simulink model "BlokRegulatoraPIDUlamkowegoRzedu"  (R2017b)
settings: Solver=VariableStepAuto  StartTime=0.0  StopTime=400  FixedStep=0.01  RelTol=1e-3  EnableMultiTasking=on
settings Model: Creator=Kuba  LastModifiedBy=Kuba
settings SolverCC: AutoInsertRateTranBlk=on
settings ConfigComp: PLC_OutputDir=Out  PLC_TargetIDE=tiaportal  PLC_GenerateReport=off  PLC_LaunchReport=off

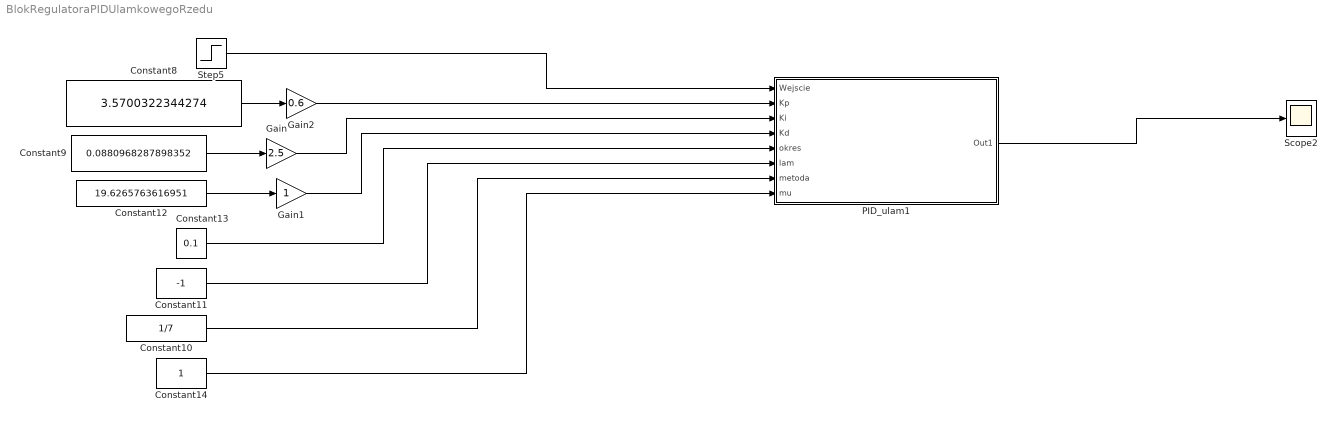
== system BlokRegulatoraPIDUlamkowegoRzedu ==
  Constant10 : Constant  Value=1/7  SampleTime=0.05
  Constant11 : Constant  Value=-1  SampleTime=0.05
  Constant12 : Constant  Value=19.6265763616951  SampleTime=0.05
  Constant13 : Constant  Value=0.1  SampleTime=0.05
  Constant14 : Constant  SampleTime=0.05
  Constant8 : Constant  Value=3.5700322344274  SampleTime=0.05
  Constant9 : Constant  Value=0.0880968287898352  SampleTime=0.05
  Gain : Gain  Gain=2.5
  Gain1 : Gain
  Gain2 : Gain  Gain=0.6
  PID_ulam1 : Subsystem  TreatAsAtomicUnit=on  SystemSampleTime=0.1
  Scope2 : Scope
  Step5 : Step  SampleTime=0.05
  wires:
  Constant10/1 -> PID_ulam1/7(metoda)
  Constant11/1 -> PID_ulam1/6(lam)
  Constant8/1 -> Gain2/1
  Constant13/1 -> PID_ulam1/5(okres)
  Constant14/1 -> PID_ulam1/8("mu ")
  Constant12/1 -> Gain1/1
  Constant9/1 -> Gain/1
  Gain/1 -> PID_ulam1/3("Ki ")
  Gain1/1 -> PID_ulam1/4("Kd ")
  Gain2/1 -> PID_ulam1/2(Kp)
  Step5/1 -> PID_ulam1/1(Wejscie)
  PID_ulam1/1(Out1) -> Scope2/1

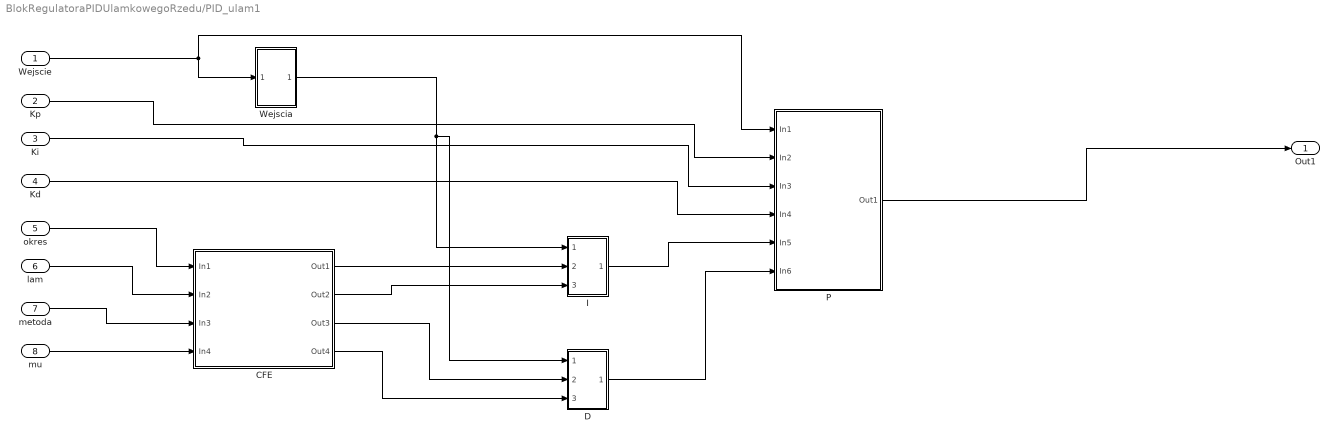
== system BlokRegulatoraPIDUlamkowegoRzedu/PID_ulam1 ==
  Wejscie : Inport
  Kp : Inport  Port=2
  "Ki " : Inport  Port=3
  "Kd " : Inport  Port=4
  okres : Inport  Port=5
  lam : Inport  Port=6
  metoda : Inport  Port=7
  "mu " : Inport  Port=8
  CFE : Subsystem  TreatAsAtomicUnit=on  SystemSampleTime=0.1
  "D " : Subsystem  TreatAsAtomicUnit=on  SystemSampleTime=0.1
  "I " : Subsystem  TreatAsAtomicUnit=on  SystemSampleTime=0.1
  "P " : Subsystem  TreatAsAtomicUnit=on  SystemSampleTime=0.1
  Wejscia : Subsystem  TreatAsAtomicUnit=on  SystemSampleTime=0.1
  Out1 : Outport
  wires:
  lam/1 -> CFE/2(In2)
  okres/1 -> CFE/1(In1)
  metoda/1 -> CFE/3(In3)
  "mu "/1 -> CFE/4(In4)
  Wejscie/1 -> "P "/1(In1), Wejscia/1(In1)
  Wejscia/1(Out1) -> "I "/1(In1), "D "/1(In1)
  CFE/3(Out3) -> "D "/2(In2)
  CFE/4(Out4) -> "D "/3(In3)
  CFE/1(Out1) -> "I "/2(In2)
  CFE/2(Out2) -> "I "/3(In3)
  Kp/1 -> "P "/2(In2)
  "Ki "/1 -> "P "/3(In3)
  "Kd "/1 -> "P "/4(In4)
  "I "/1(Out1) -> "P "/5(In5)
  "D "/1(Out1) -> "P "/6(In6)
  "P "/1(Out1) -> Out1/1

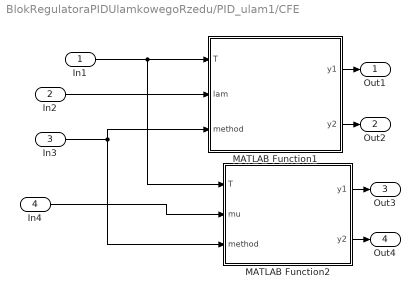
== system BlokRegulatoraPIDUlamkowegoRzedu/PID_ulam1/CFE ==
  In1 : Inport
  In2 : Inport  Port=2
  In3 : Inport  Port=3
  In4 : Inport  Port=4
  MATLAB Function1 : MATLAB Function  TreatAsAtomicUnit=on
  MATLAB Function2 : MATLAB Function  TreatAsAtomicUnit=on
  Out1 : Outport
  Out2 : Outport  Port=2
  Out3 : Outport  Port=3
  Out4 : Outport  Port=4
  wires:
  In1/1 -> MATLAB Function2/1(T), MATLAB Function1/1(T)
  In2/1 -> MATLAB Function1/2(lam)
  In3/1 -> MATLAB Function1/3(method), MATLAB Function2/3(method)
  In4/1 -> MATLAB Function2/2(mu)
  MATLAB Function1/1(y1) -> Out1/1
  MATLAB Function2/1(y1) -> Out3/1
  MATLAB Function1/2(y2) -> Out2/1
  MATLAB Function2/2(y2) -> Out4/1

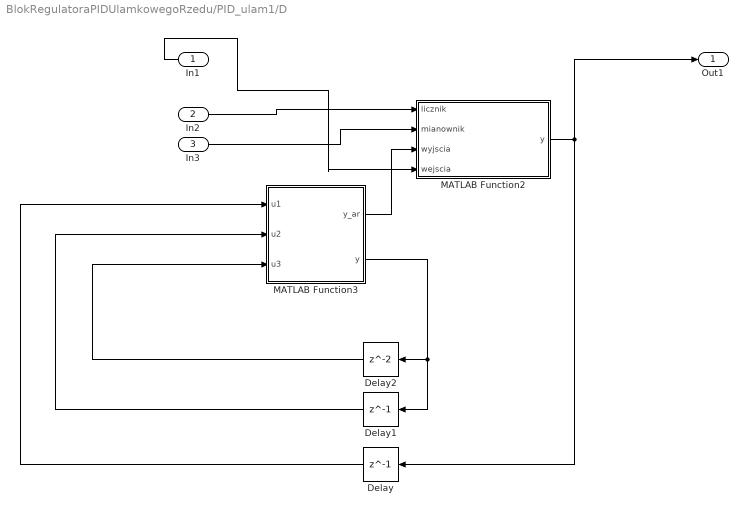
== system BlokRegulatoraPIDUlamkowegoRzedu/PID_ulam1/D  ==
  In1 : Inport
  In2 : Inport  Port=2
  In3 : Inport  Port=3
  Delay : Delay  DelayLength=1  SampleTime=0.1
  Delay1 : Delay  DelayLength=1  SampleTime=0.1
  Delay2 : Delay  SampleTime=0.1
  MATLAB Function2 : MATLAB Function  TreatAsAtomicUnit=on  SystemSampleTime=0.1
  MATLAB Function3 : MATLAB Function  TreatAsAtomicUnit=on  SystemSampleTime=0.1
  Out1 : Outport
  wires:
  In3/1 -> MATLAB Function2/2(mianownik)
  In2/1 -> MATLAB Function2/1(licznik)
  In1/1 -> MATLAB Function2/4(wejscia)
  Delay1/1 -> MATLAB Function3/2(u2)
  MATLAB Function3/2(y) -> Delay2/1, Delay1/1
  MATLAB Function3/1(y_ar) -> MATLAB Function2/3(wyjscia)
  Delay/1 -> MATLAB Function3/1(u1)
  MATLAB Function2/1(y) -> Out1/1, Delay/1
  Delay2/1 -> MATLAB Function3/3(u3)

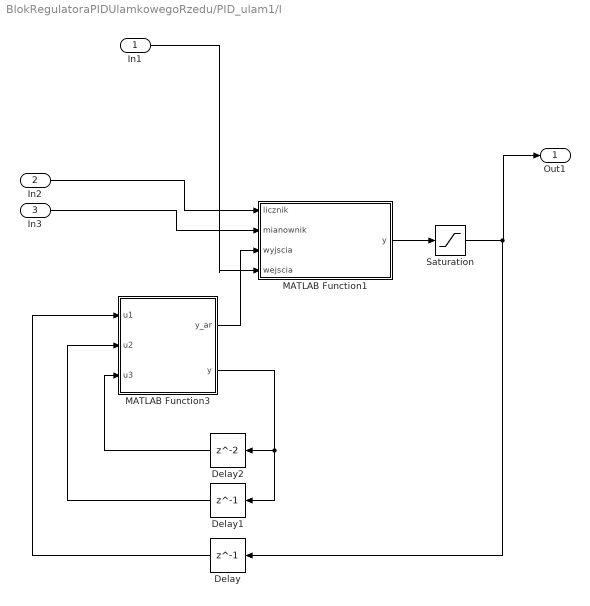
== system BlokRegulatoraPIDUlamkowegoRzedu/PID_ulam1/I  ==
  In1 : Inport
  In2 : Inport  Port=2
  In3 : Inport  Port=3
  Delay : Delay  DelayLength=1  SampleTime=0.1
  Delay1 : Delay  DelayLength=1  SampleTime=0.1
  Delay2 : Delay  SampleTime=0.1
  MATLAB Function1 : MATLAB Function  TreatAsAtomicUnit=on  SystemSampleTime=0.1
  MATLAB Function3 : MATLAB Function  TreatAsAtomicUnit=on  SystemSampleTime=0.1
  Saturation : Saturate  UpperLimit=inf  LowerLimit=-inf  LinearizeAsGain=off
  Out1 : Outport
  wires:
  In2/1 -> MATLAB Function1/1(licznik)
  In3/1 -> MATLAB Function1/2(mianownik)
  In1/1 -> MATLAB Function1/4(wejscia)
  Delay/1 -> MATLAB Function3/1(u1)
  MATLAB Function3/2(y) -> Delay2/1, Delay1/1
  Delay2/1 -> MATLAB Function3/3(u3)
  Delay1/1 -> MATLAB Function3/2(u2)
  MATLAB Function3/1(y_ar) -> MATLAB Function1/3(wyjscia)
  MATLAB Function1/1(y) -> Saturation/1
  Saturation/1 -> Delay/1, Out1/1

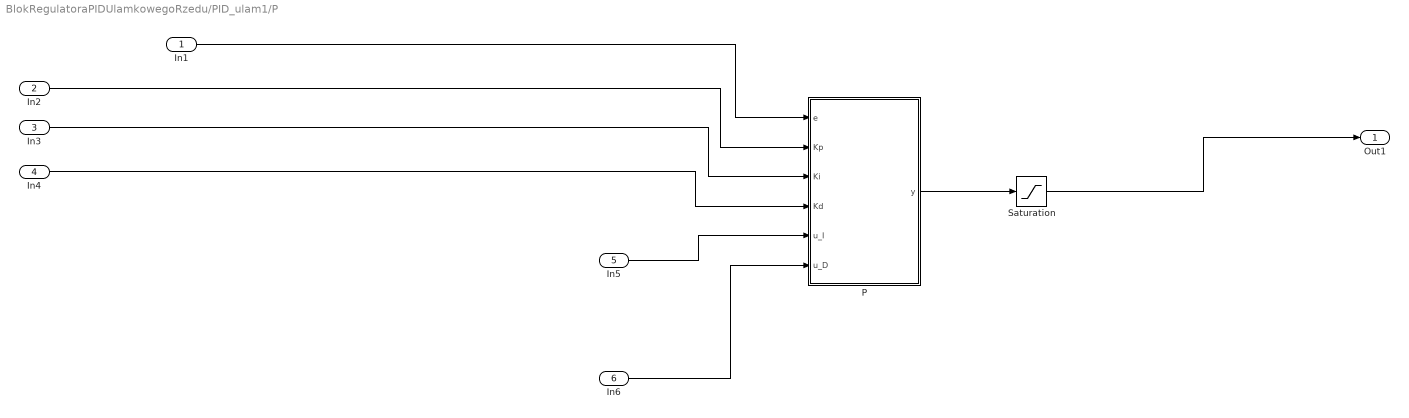
== system BlokRegulatoraPIDUlamkowegoRzedu/PID_ulam1/P  ==
  In1 : Inport
  In2 : Inport  Port=2
  In3 : Inport  Port=3
  In4 : Inport  Port=4
  In5 : Inport  Port=5
  In6 : Inport  Port=6
  "P " : MATLAB Function  TreatAsAtomicUnit=on  SystemSampleTime=0.1
  Saturation : Saturate  UpperLimit=inf  LowerLimit=-inf  LinearizeAsGain=off
  Out1 : Outport
  wires:
  In4/1 -> "P "/4(Kd)
  In2/1 -> "P "/2(Kp)
  In3/1 -> "P "/3(Ki)
  In1/1 -> "P "/1(e)
  In6/1 -> "P "/6(u_D)
  In5/1 -> "P "/5(u_I)
  "P "/1(y) -> Saturation/1
  Saturation/1 -> Out1/1

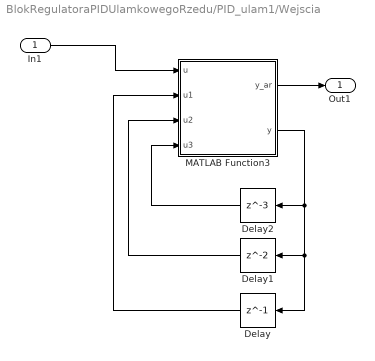
== system BlokRegulatoraPIDUlamkowegoRzedu/PID_ulam1/Wejscia ==
  In1 : Inport
  Delay : Delay  DelayLength=1  SampleTime=0.1
  Delay1 : Delay  SampleTime=0.1
  Delay2 : Delay  DelayLength=3  SampleTime=0.1
  MATLAB Function3 : MATLAB Function  TreatAsAtomicUnit=on  SystemSampleTime=0.1
  Out1 : Outport
  wires:
  Delay2/1 -> MATLAB Function3/4(u3)
  In1/1 -> MATLAB Function3/1(u)
  Delay/1 -> MATLAB Function3/2(u1)
  MATLAB Function3/2(y) -> Delay2/1, Delay1/1, Delay/1
  Delay1/1 -> MATLAB Function3/3(u2)
  MATLAB Function3/1(y_ar) -> Out1/1

== matlab function BlokRegulatoraPIDUlamkowegoRzedu/PID_ulam1/CFE/MATLAB Function1 ==
  data: y1 output; y2 output; T input; lam input; method input
function [y1,y2]= CFEI_sim(T,lam,method)

[licznik,mianownik]=CFE2(T,lam,method);

y1 = -licznik;
y2 = -mianownik;
end

== matlab function BlokRegulatoraPIDUlamkowegoRzedu/PID_ulam1/CFE/MATLAB Function2 ==
  data: T input; y1 output; mu input; method input; y2 output
function [y1,y2]= CFED_sim(T,mu,method)

[licznik,mianownik]=CFE2(T,mu,method);

y1 = licznik;
y2 = mianownik;
end

== matlab function BlokRegulatoraPIDUlamkowegoRzedu/PID_ulam1/D /MATLAB Function2 ==
  data: licznik input; y output; mianownik input; wyjscia input; wejscia input
function y = D_mu(licznik,mianownik,wyjscia,wejscia)



temp_l = (licznik.*wejscia);

temp = (mianownik.*wyjscia);


out = (1/mianownik(1))*(-sum(temp)+sum(temp_l));

y = out;

== matlab function BlokRegulatoraPIDUlamkowegoRzedu/PID_ulam1/D /MATLAB Function3 ==
  data: u1 input; u2 input; y_ar output; u3 input; y output
function [y_ar,y]= del2(u1,u2,u3)

y=u1;
y_ar = [0,u1,u2,u3];

== matlab function BlokRegulatoraPIDUlamkowegoRzedu/PID_ulam1/I /MATLAB Function1 ==
  data: licznik input; y output; mianownik input; wyjscia input; wejscia input
function y= I_lam(licznik,mianownik,wyjscia,wejscia)


temp_l = (licznik.*wejscia);

temp = (mianownik.*wyjscia);


out = (1/mianownik(1))*(-sum(temp)+sum(temp_l));



y = out;

== matlab function BlokRegulatoraPIDUlamkowegoRzedu/PID_ulam1/I /MATLAB Function3 ==
  data: u1 input; u2 input; y_ar output; u3 input; y output
function [y_ar,y]= del2(u1,u2,u3)

y=u1;
y_ar = [0,u1,u2,u3];

== matlab function BlokRegulatoraPIDUlamkowegoRzedu/PID_ulam1/P /P  ==
  data: e input; Kp input; Ki input; y output; Kd input; u_I input; u_D input
function y= P(e,Kp,Ki,Kd,u_I,u_D)



y = Kp*e+Ki*u_I+Kd*u_D;

== matlab function BlokRegulatoraPIDUlamkowegoRzedu/PID_ulam1/Wejscia/MATLAB Function3 ==
  data: y_ar output; u input; y output; u1 input; u2 input; u3 input
function [y_ar,y]= del(u,u1,u2,u3)

y=u;
y_ar = [u,u1,u2,u3];
